simulink model "sim_hinf"  (Simulink 6.2)
settings: Solver=ode45  StartTime=0.0  StopTime=1000.0  RelTol=1e-3
undefined symbols (not defined in the file or in its folder): dF, dKH2, dKinf, dKinf0, nF, nKH2, nKinf, nKinf0, T, wIn
settings Model: LastModifiedBy=Administrator
settings OptimizationCC: InlineInvariantSignals=on
settings DebuggingCC: SolverPrmCheckMsg=warning

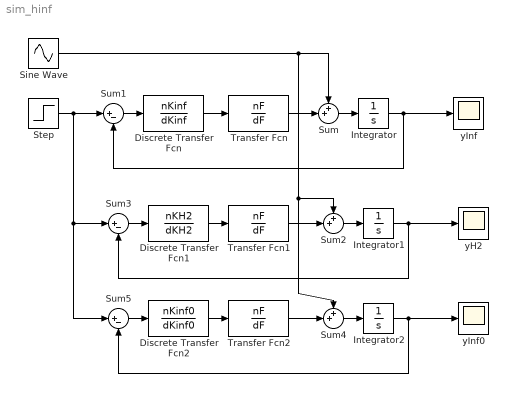
== system sim_hinf ==
  Discrete Transfer Fcn : DiscreteTransferFcn  Numerator=nKinf  Denominator=dKinf  SampleTime=T
  Discrete Transfer Fcn1 : DiscreteTransferFcn  Numerator=nKH2  Denominator=dKH2  SampleTime=T
  Discrete Transfer Fcn2 : DiscreteTransferFcn  Numerator=nKinf0  Denominator=dKinf0  SampleTime=T
  Integrator : Integrator
  Integrator1 : Integrator
  Integrator2 : Integrator
  Sine Wave : Sin  Frequency=wIn  SampleTime=0
  Step : Step  Time=0  After=0  SampleTime=0
  Sum : Sum  Inputs=++|
  Sum1 : Sum  Inputs=|+-
  Sum2 : Sum  Inputs=++|
  Sum3 : Sum  Inputs=|+-
  Sum4 : Sum  Inputs=++|
  Sum5 : Sum  Inputs=|+-
  Transfer Fcn : TransferFcn  Numerator=nF  Denominator=dF
  Transfer Fcn1 : TransferFcn  Numerator=nF  Denominator=dF
  Transfer Fcn2 : TransferFcn  Numerator=nF  Denominator=dF
  yH2 : Scope
      settings: TimeRange=500  YMin=-15  YMax=15  SaveName=yH2  DataFormat=Array
  yInf : Scope
      settings: TimeRange=500  YMin=-15  YMax=15  SaveName=yInf  DataFormat=Array
  yInf0 : Scope
      settings: TimeRange=500  YMin=-15  YMax=15  SaveName=yInf0  DataFormat=Array
  wires:
  Transfer Fcn/1 -> Sum/2
  Sum/1 -> Integrator/1
  Discrete Transfer Fcn/1 -> Transfer Fcn/1
  Step/1 -> Sum1/1, Sum3/1, Sum5/1
  Sum1/1 -> Discrete Transfer Fcn/1
  Integrator/1 -> yInf/1, Sum1/2
  Transfer Fcn1/1 -> Sum2/2
  Sum2/1 -> Integrator1/1
  Discrete Transfer Fcn1/1 -> Transfer Fcn1/1
  Sum3/1 -> Discrete Transfer Fcn1/1
  Integrator1/1 -> Sum3/2, yH2/1
  Sine Wave/1 -> Sum/1, Sum2/1, Sum4/1
  Transfer Fcn2/1 -> Sum4/2
  Sum4/1 -> Integrator2/1
  Discrete Transfer Fcn2/1 -> Transfer Fcn2/1
  Sum5/1 -> Discrete Transfer Fcn2/1
  Integrator2/1 -> yInf0/1, Sum5/2
